simulink model "drone_model"  (R2020a)
settings: Solver=VariableStepAuto  StartTime=0.0  StopTime=13  RelTol=1e-3
values from neighbouring files (symbols this model uses):
  clientID = sim.simxStart('127.0.0.1',19999,true,true,5000,5)    [initCoppelia.m]    (also in simpleTest.m = sim.simxStart('192.168.1.6',19999,true,true,5000,5))
  g = [0 0 1]'*Gr    [Kfilter.m]    (also in kalman_filter.m = [0 0 1]'*G)
  sim = remApi('remoteApi')    [initCoppelia.m]    (also in simpleTest.m)
undefined symbols (not defined in the file or in its folder): d, I, Kf, Km, m, sendCoppelia
libraries: vrlib x1, simulink x1
settings Model: Creator=roger  LastModifiedBy=roger
settings DataIOCC: ReturnWorkspaceOutputs=off

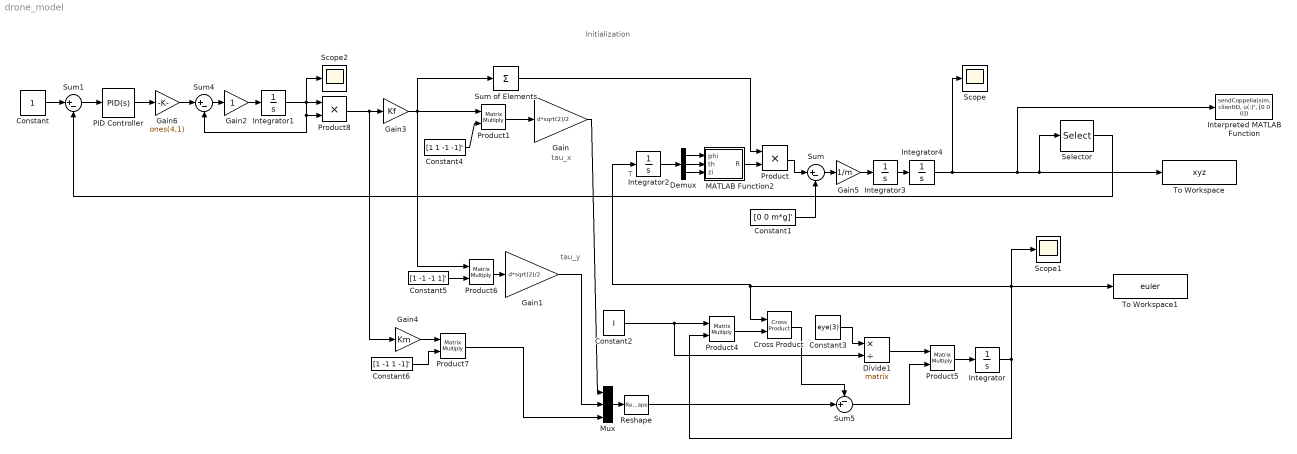
== system drone_model ==
  note: T
  note: tau_y
  note: tau_x
  note: Initialization
  Constant : Constant
  Constant1 : Constant  Value=[0 0 m*g]'  VectorParams1D=off
  Constant2 : Constant  Value=I
  Constant3 : Constant  Value=eye(3)
  Constant4 : Constant  Value=[1 1 -1 -1]'  VectorParams1D=off
  Constant5 : Constant  Value=[1 -1 -1 1]'  VectorParams1D=off
  Constant6 : Constant  Value=[1 -1 1 -1]'  VectorParams1D=off
  Cross Product : vrlib/Utilities/Cross Product
  Demux : Demux  Outputs=3
  Divide1 : Product  Inputs=*/  Multiplication=Matrix(*)
  Gain : Gain  Gain=d*sqrt(2)/2
  Gain1 : Gain  Gain=d*sqrt(2)/2
  Gain2 : Gain
  Gain3 : Gain  Gain=Kf
  Gain4 : Gain  Gain=Km
  Gain5 : Gain  Gain=1/m
  Gain6 : Gain  Gain=ones(4,1)
  Integrator{,1..4} (5 alike) : Integrator
  Interpreted MATLAB Function : MATLABFcn  MATLABFcn=sendCoppelia(sim, clientID, u(:)', [0 0 0])  OutputDimensions=0
  MATLAB Function2 : MATLAB Function  TreatAsAtomicUnit=on
  Mux : Mux  Inputs=3
  PID Controller : simulink/Continuous/PID Controller  Controller=PID  Form=Parallel  TimeDomain=Continuous-time  UseExternalTs=off  SampleTime=-1  IntegratorMethod=Forward Euler  FilterMethod=Forward Euler  ControllerParametersSource=internal  P=0.1  I=0  D=0  UseFilter=on  N=100  TunerSelectOption=Transfer Function Based (PID Tuner App)  InitialConditionSource=internal  InitialConditionForIntegrator=0  InitialConditionForFilter=0  DifferentiatorICPrevScaledInput=0  ExternalReset=none  TrackingMode=off  Kt=1  LimitOutput=off  UpperSaturationLimit=inf  LowerSaturationLimit=-inf  LinearizeAsGain=on  AntiWindupMode=none  Kb=1  POutMin=[]  POutMax=[]  IOutMin=[]  IOutMax=[]  DOutMin=[]  DOutMax=[]  NOutMin=[]  NOutMax=[]  SumOutMin=[]  SumOutMax=[]  SaturationOutMin=[]  SaturationOutMax=[]  PParamMin=[]  PParamMax=[]  IParamMin=[]  IParamMax=[]  DParamMin=[]  DParamMax=[]  NParamMin=[]  NParamMax=[]  KbParamMin=[]  KbParamMax=[]  KtParamMin=[]  KtParamMax=[]  KbOutMin=[]  KbOutMax=[]  KtOutMin=[]  KtOutMax=[]  IntegratorOutMin=[]  IntegratorOutMax=[]  FilterOutMin=[]  FilterOutMax=[]  SumI1OutMin=[]  SumI1OutMax=[]  SumI2OutMin=[]  SumI2OutMax=[]  SumI3OutMin=[]  SumI3OutMax=[]  SumI4OutMin=[]  SumI4OutMax=[]  SumDOutMin=[]  SumDOutMax=[]  DifferentiatorOutMin=[]  DifferentiatorOutMax=[]  FilterDiffOutCoefMin=[]  FilterDiffOutCoefMax=[]  ReciprocalOutMin=[]  ReciprocalOutMax=[]  SumDenOutMin=[]  SumDenOutMax=[]  SumNumOutMin=[]  SumNumOutMax=[]  DivideOutMin=[]  DivideOutMax=[]  UdiffTsProdOutMin=[]  UdiffTsProdOutMax=[]  NTsProdOutMin=[]  NTsProdOutMax=[]  UintegralTsProdOutMin=[]  UintegralTsProdOutMax=[]  UngainTsProdOutMin=[]  UngainTsProdOutMax=[]  IntegratorContinuousStateAttributes=''  IntegratorStateMustResolveToSignalObject=off  IntegratorRTWStateStorageClass=Auto  FilterContinuousStateAttributes=''  FilterStateMustResolveToSignalObject=off  FilterRTWStateStorageClass=Auto  ParallelPVariant=InternalParameters  IdealPVariant=Disabled  IVariant=InternalParameters  DVariant=InternalParameters  IntegratorVariant=Continuous  SatVariant=Disabled  AWVariant=Passthrough  PCopyVariant=Disabled  TRVariant=Disabled  FdbkBlocksVariant=Forward  IdealPFdbkVariant=Disabled  SatFdbkVariant=Disabled  DerivativeFilterVariant=ContFilter  NVariant=InternalParameters  NCopyVariant=Disabled  FilterICVariant=InternalICsFilter  IntegratorICVariant=InternalICs  ExternalResetVariant=Disabled  TRSumVariant=Passthrough  SumFdbkVariant=Disabled  SumVariant=Sum_PID  TsampFilterVariant=InternalTs  TsampNgainVariant=Passthrough  TsampIntegralVariant=Passthrough
  Product : Product
  Product{1,4..7} (5 alike) : Product  Multiplication=Matrix(*)
  Product8 : Product
  Reshape : Reshape  OutputDimensionality=Column vector (2-D)
  Scope : Scope
  Scope1 : Scope
  Scope2 : Scope
  Selector : Selector  InputPortWidth=3  IndexOptions=Index vector (dialog)  Indices=[3]  OutputSizes=1
  Sum : Sum  Inputs=|+-
  Sum of Elements : Sum  Inputs=+
  Sum1 : Sum  Inputs=|+-
  Sum4 : Sum  Inputs=|+-
  Sum5 : Sum  Inputs=-+|
  To Workspace : ToWorkspace  VariableName=xyz  SaveFormat=Timeseries  SampleTime=-1
  To Workspace1 : ToWorkspace  VariableName=euler  SaveFormat=Timeseries  SampleTime=-1
  wires:
  Product1/1 -> Gain/1
  Product6/1 -> Gain1/1
  Gain/1 -> Mux/1
  Gain1/1 -> Mux/2
  Constant2/1 -> Divide1/2, Product4/1
  Product4/1 -> Cross Product/2
  Mux/1 -> Reshape/1
  Constant3/1 -> Divide1/1
  Product5/1 -> Integrator/1
  Integrator/1 -> Product4/2, To Workspace1/1, Scope1/1, Integrator2/1, Cross Product/1
  Divide1/1 -> Product5/1
  Sum5/1 -> Product5/2
  Reshape/1 -> Sum5/2
  Cross Product/1 -> Sum5/1
  PID Controller/1 -> Gain6/1
  Sum4/1 -> Gain2/1
  Gain2/1 -> Integrator1/1
  Constant4/1 -> Product1/2
  Constant5/1 -> Product6/2
  Integrator1/1 -> Scope2/1, Product8/2, Sum4/2, Product8/1
  Constant6/1 -> Product7/2
  Product7/1 -> Mux/3
  Product8/1 -> Gain4/1, Gain3/1
  Gain3/1 -> Product6/1, Sum of Elements/1, Product1/1
  Gain4/1 -> Product7/1
  Integrator2/1 -> Demux/1
  Demux/1 -> MATLAB Function2/1(phi)
  Demux/2 -> MATLAB Function2/2(th)
  Demux/3 -> MATLAB Function2/3(zi)
  Product/1 -> Sum/1
  Constant1/1 -> Sum/2
  Sum/1 -> Gain5/1
  Gain5/1 -> Integrator3/1
  Integrator3/1 -> Integrator4/1
  Integrator4/1 -> Scope/1, Interpreted MATLAB Function/1, Selector/1, To Workspace/1
  MATLAB Function2/1(R) -> Product/2
  Sum of Elements/1 -> Product/1
  Sum1/1 -> PID Controller/1
  Selector/1 -> Sum1/2
  Constant/1 -> Sum1/1
  Gain6/1 -> Sum4/1

== matlab function drone_model/MATLAB Function2 ==
  data: phi input; th input; zi input; R output
function R = rotz(phi, th, zi)
R = [cos(zi)*sin(th)+cos(th)*sin(phi)*sin(zi); ...
    sin(zi)*sin(th) - cos(zi)*cos(th)*sin(phi);...
    cos(phi)*cos(th)];
end
